simulink model "Subsystem0"  (R2020b)
settings: Solver=FixedStepAuto  StartTime=0.0  StopTime=10.0  FixedStep=0.2  RelTol=1e-3
settings Model: Creator=Aradhana desai  LastModifiedBy=Aradhana desai
settings DataIOCC: SaveOutput=off  SaveTime=off

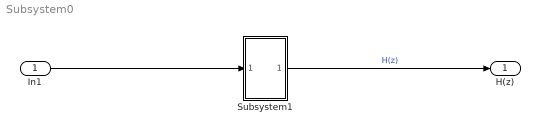
== system Subsystem0 ==
  In1 : Inport  OutDataTypeStr=double  PortDimensions=1  SampleTime=[0,1]
  Subsystem1 : Subsystem
  H(z) : Outport  OutDataTypeStr=double  PortDimensions=1  SampleTime=[0.20000000000000001,0]
  wires:
  Subsystem1/1(H(z)) -> H(z)/1  "H(z)"
  In1/1 -> Subsystem1/1(In1)

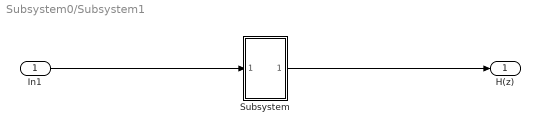
== system Subsystem0/Subsystem1 ==
  In1 : Inport
  Subsystem : Subsystem  TreatAsAtomicUnit=on
  H(z) : Outport
  wires:
  Subsystem/1(H(z)) -> H(z)/1
  In1/1 -> Subsystem/1(In1)

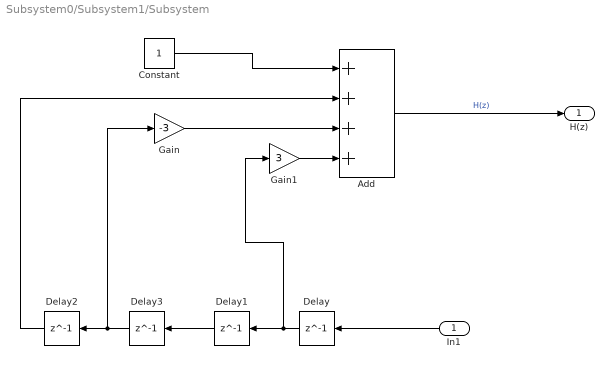
== system Subsystem0/Subsystem1/Subsystem ==
  In1 : Inport
  Add : Sum  Inputs=++++
  Constant : Constant
  Delay{,1..3} (4 alike) : Delay  DelayLength=1
  Gain : Gain  Gain=-3
  Gain1 : Gain  Gain=3
  H(z) : Outport
  wires:
  Gain1/1 -> Add/4
  Delay1/1 -> Delay3/1
  Delay2/1 -> Add/2
  Gain/1 -> Add/3
  Add/1 -> H(z)/1  "H(z)"
  Constant/1 -> Add/1
  Delay3/1 -> Delay2/1, Gain/1
  Delay/1 -> Delay1/1, Gain1/1
  In1/1 -> Delay/1
